simulink model "Super4_tmp"  (Simulink 8.3)
settings: Solver=ode45  StartTime=0.0  StopTime=10.0  RelTol=1e-3
settings Model: Creator=scaife  LastModifiedBy=bourbouh  CovSFcnEnable=on  ExtModeAutoUpdateStatusClock=off
settings DataIOCC: SignalLoggingName=sigsOut
settings DebuggingCC: SaveWithParameterizedLinksMsg=none  SignalResolutionControl=TryResolveAllWithWarning  SolverPrmCheckMsg=none  MultiTaskDSMMsg=warning  MultiTaskCondExecSysMsg=none  FrameProcessingCompatibilityMsg=error  StateNameClashWarn=none  StrictBusMsg=None
settings HardwareCC: TargetUnknown=on
settings SFSimCC: SimParseCustomCode=off
settings GRTTargetCC: GeneratePreprocessorConditionals=Use local settings

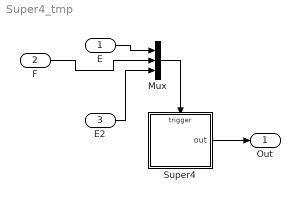
== system Super4_tmp ==
  E : Inport
  F : Inport  Port=2
  E2 : Inport  Port=3
  Mux : Mux  Inputs=3
  Super4 : Stateflow chart  TreatAsAtomicUnit=on
      settings: PermitHierarchicalResolution=ParametersOnly
  Out : Outport
  wires:
  Super4/1(out) -> Out/1
  E/1 -> Mux/1
  F/1 -> Mux/2
  E2/1 -> Mux/3
  Mux/1 -> Super4/Trigger

== stateflow chart Super4 ==
  state A
    du : out++;
    state A1
      du : out++;
    (default) -> A1
  state B
    du : out++;
    state B1
      du : out++;
    (default) -> B1
  state C
    du : out++;
  state D
    du : out++;
  C -> D [order 1] : F
  (default) -> C
  A -> B : G
  B1 -> D [order 1] : E
  A1 -> B1 [order 1] : E
  C -> A1 [order 2] : E
  A1 -> C [order 2] : F
  D -> B1 [order 2] : F
  B1 -> A1 [order 2] : F
  D -> C [order 1] : E
  B -> A : G
  data: out output double
  events: E input EITHER_EDGE_EVENT; G input EITHER_EDGE_EVENT; F input EITHER_EDGE_EVENT
